simulink model "rotatedQpskFFRC"  (R2015a)
settings: Solver=ode45  StartTime=0.0  StopTime=Inf  RelTol=1e-3
libraries: commblkintrlv2 x6, commnoisgen2 x2, commsink2 x1, commchan3 x1, commrandsrc2 x1, commdigbbndpm3 x1
settings Model: Creator=konstantis  LastModifiedBy=konstantis

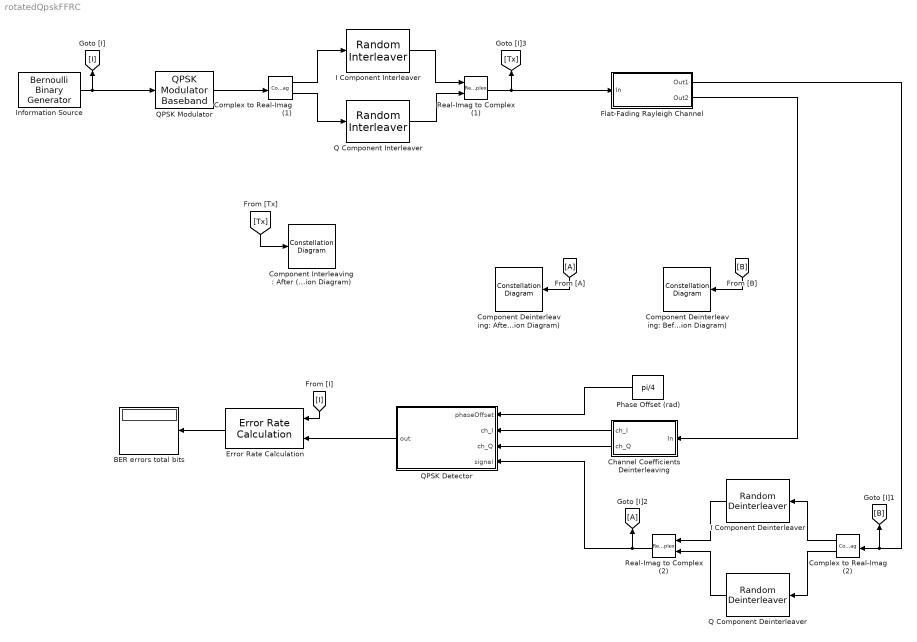
== system rotatedQpskFFRC ==
  BER errors total bits : Display
      settings: Format=short_e
  Channel Coefficients Deinterleaving : Subsystem
  Complex to Real-Imag (1) : ComplexToRealImag
  Complex to Real-Imag (2) : ComplexToRealImag
  Component Deinterleaving: After (Constellation Diagram) : ConstellationDiagram
  Component Deinterleaving: Before (Constellation Diagram) : ConstellationDiagram
  Component Interleaving: After (Constellation Diagram) : ConstellationDiagram
  Error Rate Calculation : commsink2/Error Rate Calculation  N=0  st_delay=0  cp_mode=Entire frame  subframe=[]  PMode=Port  WsName=ErrorVec  RsMode2=off  stop=off  numErr=100  maxBits=1e6
  Flat-Fading Rayleigh Channel : Subsystem
  I Component Deinterleaver : commblkintrlv2/Random Deinterleaver  N=500  seed=12345
  I Component Interleaver : commblkintrlv2/Random Interleaver  N=500  seed=12345
  Information Source : commrandsrc2/Bernoulli Binary Generator  P=0.5  seed=61  Ts=.001  frameBased=on  sampPerFrame=1000  orient=off  outDataType=double
  Phase Offset (rad) : Constant  Value=pi/4
  Q Component Deinterleaver : commblkintrlv2/Random Deinterleaver  N=500  seed=54321
  Q Component Interleaver : commblkintrlv2/Random Interleaver  N=500  seed=54321
  QPSK Detector : MATLAB Function  TreatAsAtomicUnit=on
  QPSK Modulator : commdigbbndpm3/QPSK Modulator Baseband  InType=Bit  Enc=Gray  Ph=pi/4  outDtype=double  outWordLen=16  outUDDataType=sfix(16)  outFracLenMode=Best precision  outFracLen=15
  Real-Imag to Complex (1) : RealImagToComplex
  Real-Imag to Complex (2) : RealImagToComplex
  wires:
  Information Source/1 -> QPSK Modulator/1, [I]
  QPSK Modulator/1 -> Complex to Real-Imag (1)/1
  Real-Imag to Complex (1)/1 -> Flat-Fading Rayleigh Channel/1(In), [Tx]
  Error Rate Calculation/1 -> BER errors total bits/1
  Flat-Fading Rayleigh Channel/1(Out1) -> [B], Complex to Real-Imag (2)/1
  Real-Imag to Complex (2)/1 -> [A], QPSK Detector/4(signal)
  QPSK Detector/1(out) -> Error Rate Calculation/2
  Complex to Real-Imag (1)/1 -> I Component Interleaver/1
  I Component Interleaver/1 -> Real-Imag to Complex (1)/1
  Complex to Real-Imag (1)/2 -> Q Component Interleaver/1
  Q Component Interleaver/1 -> Real-Imag to Complex (1)/2
  Complex to Real-Imag (2)/1 -> I Component Deinterleaver/1
  I Component Deinterleaver/1 -> Real-Imag to Complex (2)/1
  Complex to Real-Imag (2)/2 -> Q Component Deinterleaver/1
  Q Component Deinterleaver/1 -> Real-Imag to Complex (2)/2
  Flat-Fading Rayleigh Channel/2(Out2) -> Channel Coefficients Deinterleaving/1(In)
  Phase Offset (rad)/1 -> QPSK Detector/1(phaseOffset)
  [I] -> Error Rate Calculation/1
  Channel Coefficients Deinterleaving/1(ch_I) -> QPSK Detector/2(ch_I)
  Channel Coefficients Deinterleaving/2(ch_Q) -> QPSK Detector/3(ch_Q)
  [B] -> Component Deinterleaving: Before (Constellation Diagram)/1
  [A] -> Component Deinterleaving: After (Constellation Diagram)/1
  [Tx] -> Component Interleaving: After (Constellation Diagram)/1

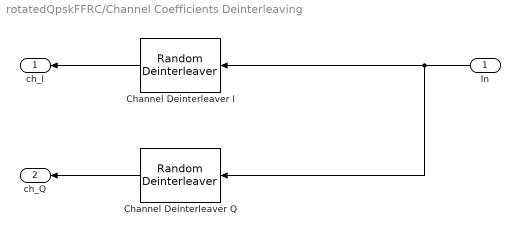
== system rotatedQpskFFRC/Channel Coefficients Deinterleaving ==
  In : Inport
  Channel Deinterleaver I : commblkintrlv2/Random Deinterleaver  N=500  seed=12345
  Channel Deinterleaver Q : commblkintrlv2/Random Deinterleaver  N=500  seed=54321
  ch_I : Outport
  ch_Q : Outport  Port=2
  wires:
  In/1 -> Channel Deinterleaver Q/1, Channel Deinterleaver I/1
  Channel Deinterleaver I/1 -> ch_I/1
  Channel Deinterleaver Q/1 -> ch_Q/1

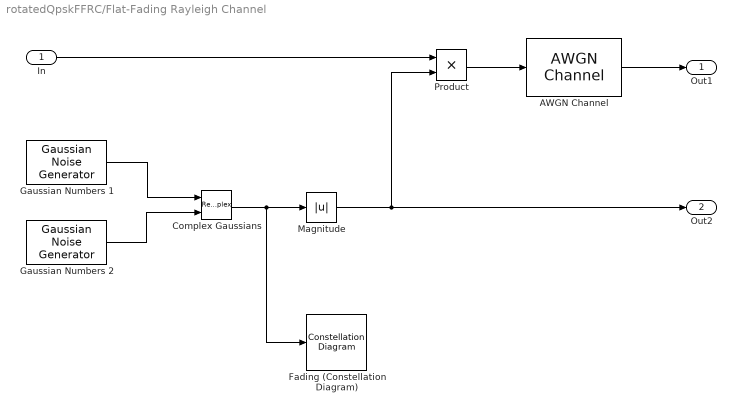
== system rotatedQpskFFRC/Flat-Fading Rayleigh Channel ==
  In : Inport
  AWGN Channel : commchan3/AWGN Channel  InputProcessing=Columns as channels (frame based)  seed=67  noiseMode="Signal to noise ratio  (SNR)"  EbNodB=10  EsNodB=10  SNRdB=23  bitsPerSym=1  Ps=1  Tsym=1  variance=1
  Complex Gaussians : RealImagToComplex
  Fading (Constellation Diagram) : ConstellationDiagram
  Gaussian Numbers 1 : commnoisgen2/Gaussian Noise Generator  m=0  d=1/2  s=41  Ts=.001  frameBased=on  sampPerFrame=500  orient=off  outDataType=double
  Gaussian Numbers 2 : commnoisgen2/Gaussian Noise Generator  m=0  d=1/2  s=410000001  Ts=.001  frameBased=on  sampPerFrame=500  orient=off  outDataType=double
  Magnitude : Abs
  Product : Product
  Out1 : Outport
  Out2 : Outport  Port=2
  wires:
  Gaussian Numbers 1/1 -> Complex Gaussians/1
  Gaussian Numbers 2/1 -> Complex Gaussians/2
  In/1 -> Product/1
  Product/1 -> AWGN Channel/1
  AWGN Channel/1 -> Out1/1
  Complex Gaussians/1 -> Magnitude/1, Fading (Constellation Diagram)/1
  Magnitude/1 -> Product/2, Out2/1

== matlab function rotatedQpskFFRC/QPSK Detector ==
  data: phaseOffset input; ch_I input; ch_Q input; out output; signal input
function out = fcn(phaseOffset, ch_I, ch_Q, signal)

% QPSK constellation
ss = [cos(phaseOffset)        + 1i * sin(phaseOffset);
      cos(phaseOffset+pi/2)   + 1i * sin(phaseOffset+pi/2);
      cos(phaseOffset+pi)     + 1i * sin(phaseOffset+pi);
      cos(phaseOffset+3*pi/2) + 1i * sin(phaseOffset+3*pi/2)];

t = zeros(2*length(signal),1);

j = 1;
for i = 1 : length(signal)
    
    % metric minimization
    [~,I] = min(abs(signal(i) - ch_I(i)*real(ss) - ch_Q(i)*1i*imag(ss)));
    
    % detection
    switch I
        case 1
            t(j,1) = 0;
            j = j + 1;
            t(j,1) = 0;
            j = j + 1;
            
        case 2
            t(j,1) = 0;
            j = j + 1;
            t(j,1) = 1;
            j = j + 1;
            
        case 3
            t(j,1) = 1;
            j = j + 1;
            t(j,1) = 1;
            j = j + 1; 
            
        otherwise
            t(j,1) = 1;
            j = j + 1;
            t(j,1) = 0;
            j = j + 1; 
    end
end
out = t;
